simulink model "regen"  (R2024b)
settings: Solver=VariableStepAuto  StartTime=0.0  StopTime=10  FixedStep=0.001  RelTol=1e-3
settings Model: Creator=Isaac  LastModifiedBy=isaac

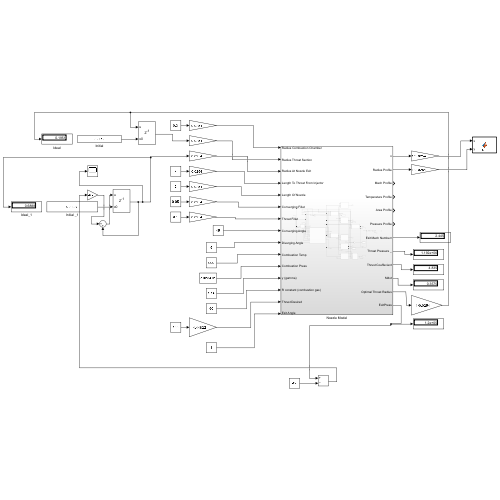
[thumbnail: Simulink's stored preview of the top-level diagram]
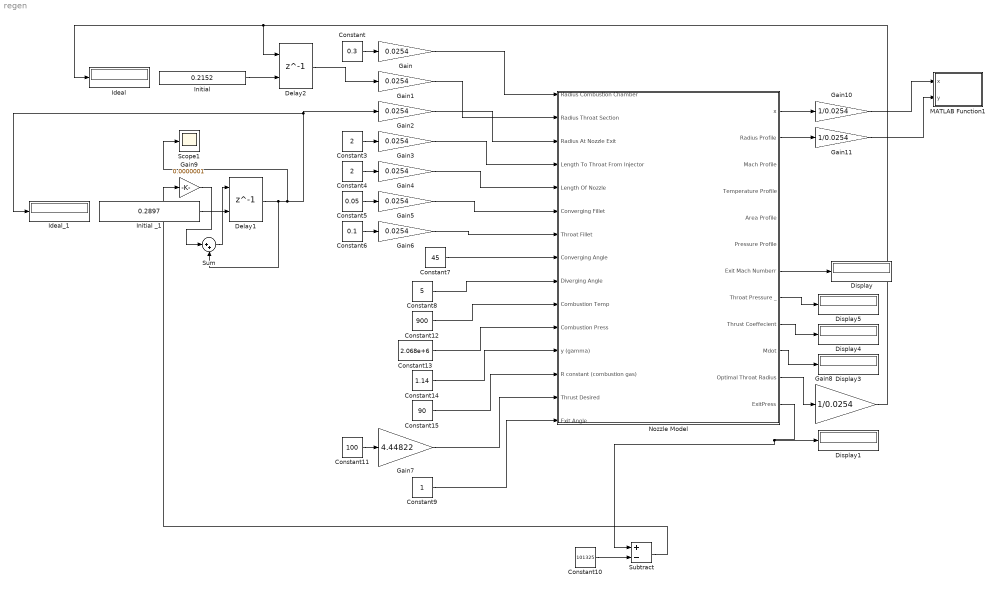
== system regen ==
  Constant : Constant  Value=0.3
  Constant10 : Constant  Value=101325
  Constant11 : Constant  Value=100
  Constant12 : Constant  Value=900
  Constant13 : Constant  Value=2.068e+6
  Constant14 : Constant  Value=1.14
  Constant15 : Constant  Value=90
  Constant3 : Constant  Value=2
  Constant4 : Constant  Value=2
  Constant5 : Constant  Value=0.05
  Constant6 : Constant  Value=0.1
  Constant7 : Constant  Value=45
  Constant8 : Constant  Value=5
  Constant9 : Constant
  Delay1 : Delay  DelayLength=1  InitialConditionSource=Input port
      settings: InputPortMap=u0,p4
  Delay2 : Delay  DelayLength=1  InitialConditionSource=Input port
      settings: InputPortMap=u0,p4
  Display{,1,3..5} (5 alike) : Display
  Gain{,1..6} (7 alike) : Gain  Gain=0.0254
  Gain10 : Gain  Gain=1/0.0254
  Gain11 : Gain  Gain=1/0.0254
  Gain7 : Gain  Gain=4.44822
  Gain8 : Gain  Gain=1/0.0254
  Gain9 : Gain  Gain=0.0000001
  Ideal : Display
  Ideal_1 : Display
  Initial : Constant  Value=0.2152
  Initial _1 : Constant  Value=0.2897
  MATLAB Function1 : MATLAB Function  TreatAsAtomicUnit=on
  Nozzle Model : Subsystem
  Scope1 : Scope
  Subtract : Sum  Inputs=+-
  Sum : Sum  Inputs=|++
  wires:
  Constant13/1 -> Nozzle Model/11(Combustion Press)
  Constant11/1 -> Gain7/1
  Constant12/1 -> Nozzle Model/10(Combustion Temp)
  Constant/1 -> Gain/1
  Constant14/1 -> Nozzle Model/12(y (gamma))
  Constant4/1 -> Gain4/1
  Constant6/1 -> Gain6/1
  Constant15/1 -> Nozzle Model/13(R constant (combustion gas))
  Constant7/1 -> Nozzle Model/8(Converging Angle)
  Constant3/1 -> Gain3/1
  Constant5/1 -> Gain5/1
  Gain4/1 -> Nozzle Model/5(Length Of Nozzle)
  Gain/1 -> Nozzle Model/1(Radius Combustion Chamber)
  Gain2/1 -> Nozzle Model/3(Radius At Nozzle Exit)
  Gain3/1 -> Nozzle Model/4(Length To Throat From Injector)
  Gain5/1 -> Nozzle Model/6(Converging Fillet)
  Gain6/1 -> Nozzle Model/7(Throat Fillet)
  Constant8/1 -> Nozzle Model/9(Diverging Angle)
  Gain7/1 -> Nozzle Model/14(Thrust Desired)
  Constant9/1 -> Nozzle Model/15(Exit Angle)
  Nozzle Model/11(Optimal Throat Radius) -> Gain8/1
  Nozzle Model/7(Exit Mach Numberr) -> Display/1
  Nozzle Model/12(ExitPress) -> Subtract/1, Display1/1
  Nozzle Model/8(Throat Pressure _) -> Display5/1
  Nozzle Model/9(Thrust Coeffecient) -> Display4/1
  Nozzle Model/10(Mdot) -> Display3/1
  Gain8/1 -> Delay2/1, Ideal/1
  Gain1/1 -> Nozzle Model/2(Radius Throat Section)
  Delay1/1 -> Sum/2, Ideal_1/1, Gain2/1, Scope1/1
  Gain9/1 -> Sum/1
  Constant10/1 -> Subtract/2
  Subtract/1 -> Gain9/1
  Sum/1 -> Delay1/1
  Initial _1/1 -> Delay1/2
  Initial/1 -> Delay2/2
  Delay2/1 -> Gain1/1
  Nozzle Model/1(x) -> Gain10/1
  Gain10/1 -> MATLAB Function1/1(x)
  Nozzle Model/2(Radius Profile) -> Gain11/1
  Gain11/1 -> MATLAB Function1/2(y)

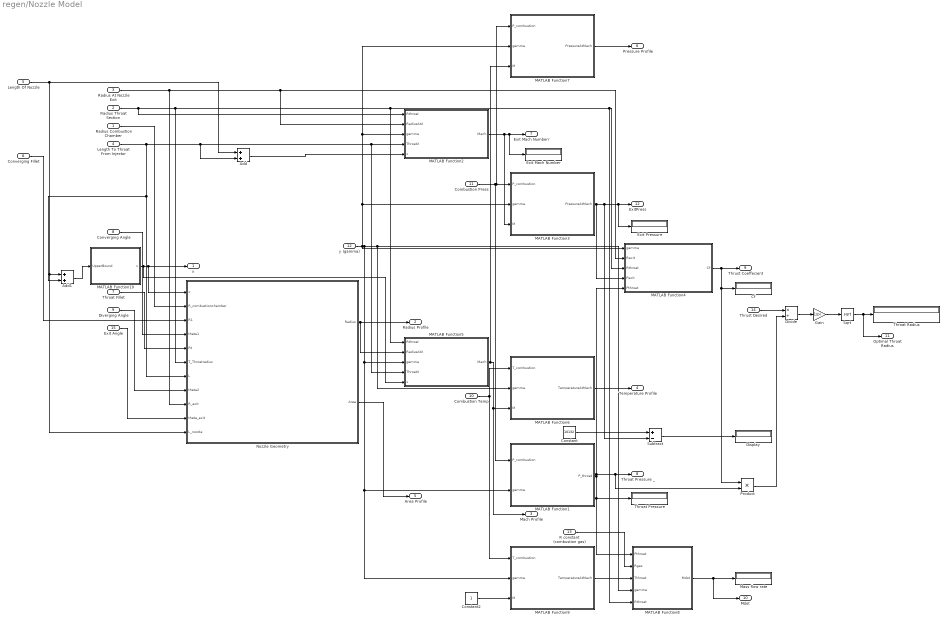
== system regen/Nozzle Model ==
  Radius Combustion Chamber : Inport
  Radius Throat Section : Inport  Port=2
  Radius At Nozzle Exit : Inport  Port=3
  Length To Throat From Injector : Inport  Port=4
  Length Of Nozzle : Inport  Port=5
  Converging Fillet : Inport  Port=6
  Throat Fillet : Inport  Port=7
  Converging Angle : Inport  Port=8
  Diverging Angle : Inport  Port=9
  Combustion Temp : Inport  Port=10
  Combustion Press : Inport  Port=11
  y (gamma) : Inport  Port=12
  R constant (combustion gas) : Inport  Port=13
  Thrust Desired : Inport  Port=14
  Exit Angle : Inport  Port=15
  Add : Sum
  Add1 : Sum
  Cf : Display
  Constant : Constant  Value=10132
  Constant2 : Constant
  Display : Display
  Divide : Product  Inputs=*/
  Exit Mach Number : Display
  Exit Pressure : Display
  Gain : Gain  Gain=1/pi
  MATLAB Function1 : MATLAB Function  TreatAsAtomicUnit=on
  MATLAB Function10 : MATLAB Function  TreatAsAtomicUnit=on
  MATLAB Function2 : MATLAB Function  TreatAsAtomicUnit=on
  MATLAB Function3 : MATLAB Function  TreatAsAtomicUnit=on
  MATLAB Function4 : MATLAB Function  TreatAsAtomicUnit=on
  MATLAB Function5 : MATLAB Function  TreatAsAtomicUnit=on
  MATLAB Function6 : MATLAB Function  TreatAsAtomicUnit=on
  MATLAB Function7 : MATLAB Function  TreatAsAtomicUnit=on
  MATLAB Function8 : MATLAB Function  TreatAsAtomicUnit=on
  MATLAB Function9 : MATLAB Function  TreatAsAtomicUnit=on
  Mass flow rate : Display
  Nozzle Geometry : MATLAB Function  TreatAsAtomicUnit=on
  Product : Product
  Sqrt : Sqrt
  Subtract : Sum  Inputs=+-
  Throat Pressure : Display
  Throat Radius : Display
  x : Outport
  Radius Profile : Outport  Port=2
  Mach Profile : Outport  Port=3
  Temperature Profile : Outport  Port=4
  Area Profile : Outport  Port=5
  Pressure Profile : Outport  Port=6
  Exit Mach Numberr : Outport  Port=7
  Throat Pressure _ : Outport  Port=8
  Thrust Coeffecient : Outport  Port=9
  Mdot : Outport  Port=10
  Optimal Throat Radius : Outport  Port=11
  ExitPress : Outport  Port=12
  wires:
  Combustion Temp/1 -> MATLAB Function6/1(T_combustion), MATLAB Function9/1(T_combustion)
  Converging Angle/1 -> Nozzle Geometry/4(theta1)
  Converging Fillet/1 -> Nozzle Geometry/3(R1)
  Length To Throat From Injector/1 -> MATLAB Function5/4(ThroatX), MATLAB Function2/4(ThroatX), Add/2, Add1/2, Nozzle Geometry/7(L)
  Combustion Press/1 -> MATLAB Function3/1(P_combustion), MATLAB Function7/1(P_combustion), MATLAB Function1/1(P_combustion)
  Diverging Angle/1 -> Nozzle Geometry/8(theta2)
  Throat Fillet/1 -> Nozzle Geometry/5(Rt)
  Length Of Nozzle/1 -> Add1/1, Nozzle Geometry/11(L_nozzle), Add/1
  Thrust Desired/1 -> Divide/1
  y (gamma)/1 -> MATLAB Function1/2(gamma), MATLAB Function9/2(gamma), MATLAB Function5/3(gamma), MATLAB Function6/2(gamma), MATLAB Function8/4(gamma), MATLAB Function7/2(gamma), MATLAB Function2/3(gamma), MATLAB Function3/2(gamma), MATLAB Function4/1(gamma)
  Add/1 -> MATLAB Function2/5(x)
  Divide/1 -> Gain/1
  Product/1 -> Divide/2
  Constant/1 -> Subtract/1
  Add1/1 -> MATLAB Function10/1(UpperBound)
  Radius At Nozzle Exit/1 -> MATLAB Function2/2(RadiusAtX), MATLAB Function4/2(Rexit), Nozzle Geometry/9(R_exit)
  Radius Combustion Chamber/1 -> Nozzle Geometry/2(R_combustionchamber)
  Radius Throat Section/1 -> MATLAB Function8/5(Rthroat), MATLAB Function4/3(Rthroat), MATLAB Function5/1(Rthroat), Nozzle Geometry/6(T_Throatradius), MATLAB Function2/1(Rthroat)
  MATLAB Function10/1(x) -> x/1, Nozzle Geometry/1(x), MATLAB Function5/5(x)
  R constant (combustion gas)/1 -> MATLAB Function8/2(Rgas)
  Exit Angle/1 -> Nozzle Geometry/10(theta_exit)
  Nozzle Geometry/1(Radius) -> Radius Profile/1, MATLAB Function5/2(RadiusAtX)
  Nozzle Geometry/2(Area) -> Area Profile/1
  MATLAB Function2/1(Mach) -> Exit Mach Numberr/1, Exit Mach Number/1, MATLAB Function3/3(M)
  Sqrt/1 -> Throat Radius/1, Optimal Throat Radius/1
  MATLAB Function5/1(Mach) -> Mach Profile/1, MATLAB Function6/3(M), MATLAB Function7/3(M)
  Constant2/1 -> MATLAB Function9/3(M)
  MATLAB Function7/1(PressureAtMach) -> Pressure Profile/1
  MATLAB Function3/1(PressureAtMach) -> ExitPress/1, Exit Pressure/1, Subtract/2, MATLAB Function4/4(Pexit)
  MATLAB Function6/1(TemperatureAtMach) -> Temperature Profile/1
  Gain/1 -> Sqrt/1
  MATLAB Function1/1(P_throat) -> Product/2, Throat Pressure _/1, MATLAB Function4/5(Pthroat), MATLAB Function8/1(Pthroat), Throat Pressure/1
  MATLAB Function9/1(TemperatureAtMach) -> MATLAB Function8/3(Tthroat)
  MATLAB Function4/1(Cf) -> Product/1, Cf/1, Thrust Coeffecient/1
  Subtract/1 -> Display/1
  MATLAB Function8/1(Mdot) -> Mass flow rate/1, Mdot/1

== matlab function regen/Nozzle Model/MATLAB Function8 ==
  data: Pthroat input; Mdot output; Rgas input; Tthroat input; gamma input; Rthroat input
function Mdot = MassFlow(Pthroat, Rgas, Tthroat, gamma, Rthroat)

Mdot = Pthroat * (Rgas * Tthroat)^-1 * sqrt(gamma * Rgas * Tthroat) * pi * Rthroat^2;

== matlab function regen/Nozzle Model/MATLAB Function9 ==
  data: T_combustion input; TemperatureAtMach output; gamma input; M input
function TemperatureAtMach = IsentropicTemperature(T_combustion, gamma, M)


TemperatureAtMach = T_combustion * (1 + 0.5*(gamma-1)*M^2)^(-1);

== matlab function regen/Nozzle Model/MATLAB Function10 ==
  data: x output size=[1 10000]; UpperBound input
function x = Span(UpperBound)

x = linspace(0, UpperBound, 10000);

== matlab function regen/MATLAB Function1 ==
  data: x input; y input
function fcn(x, y)
hold on
plot(x,y)
axis('equal')
grid on
end

== matlab function regen/Nozzle Model/Nozzle Geometry ==
  data: x input; R_combustionchamber input; R1 input; theta1 input; Rt input; T_Throatradius input; L input; theta2 input; Radius output size=[1 10000]; R_exit input; theta_exit input; L_nozzle input; Area output size=[1 10000]
function [Radius, Area] = combustionChamberProfile(x, R_combustionchamber, R1, theta1, Rt, T_Throatradius, L, theta2, R_exit, theta_exit, L_nozzle)
    y = zeros(1, length(x));
    for i=1:length(y)
    % Calculate the boundaries for each piece of the function
    boundary1 = -R1 * tan((theta1 * pi / 180) / 2) + (1 / tan(-theta1 * pi / 180)) * (R_combustionchamber + sqrt(Rt^2 - (Rt * sin(theta1 * pi / 180))^2) - T_Throatradius - Rt) + (L - Rt * sin(theta1 * pi / 180));
    
    boundary2 = boundary1 + R1 * sin(theta1 * pi / 180);
    
    boundary3 = L - Rt * sin(theta1 * pi / 180);
    
    boundary4 = L + Rt * sin(theta2 * pi / 180);
    
    exitslope = tan(theta_exit * pi / 180);

    enterslope = tan(theta2 * pi / 180);
    
    XX = [L + Rt * sin(theta2 * pi / 180), L_nozzle + L];
    YY = [-sqrt(Rt^2 - (boundary4 - L)^2) + T_Throatradius + Rt, R_exit];

    nozzleexit = spline(XX, [enterslope YY exitslope]);
    

    % Determine which piece of the function to use based on the value of x
    if x(i) >= 0 && x(i) <= boundary1
        % First piece: y = R_combustionchamber
        y(i) = R_combustionchamber;
    elseif x(i) > boundary1 && x(i) <= boundary2
        % Second piece: y = sqrt(R1^2 - (x - boundary1)^2) + R_combustionchamber - R1
        y(i) = sqrt(R1^2 - (x(i) - boundary1)^2) + R_combustionchamber - R1;
    elseif x(i) > boundary3 && x(i) <= boundary4
        % Third piece: y = -sqrt(Rt^2 - (x - L)^2) + T_Throatradius + Rt
        y(i) = -sqrt(Rt^2 - (x(i) - L)^2) + T_Throatradius + Rt;
    elseif x(i) > boundary2 && x(i) <= boundary3
        % Fourth piece: y = tan(-theta1 * pi / 180) * (x - (L - Rt * sin(theta1 * pi / 180))) - sqrt(Rt^2 - (Rt * sin(theta1 * pi / 180))^2) + T_Throatradius + Rt
        y(i) = tan(-theta1 * pi / 180) * (x(i) - (L - Rt * sin(theta1 * pi / 180))) - sqrt(Rt^2 - (Rt * sin(theta1 * pi / 180))^2) + T_Throatradius + Rt;
    elseif x(i) > boundary4 && x(i) <= XX(2)
        y(i) = ppval(nozzleexit, x(i));
    else
        % If x is outside the defined domain, return NaN (Not a Number)
        y(i) = NaN;
    end
    end

    Radius = y;
    Area = pi .* y.^2;
end

== matlab function regen/Nozzle Model/MATLAB Function1 ==
  data: P_combustion input; P_throat output; gamma input
function P_throat = ComputeThroatPressure(P_combustion, gamma)


P_throat = P_combustion*((0.5*gamma + 0.5)^((-gamma)/(gamma-1)));

== matlab function regen/Nozzle Model/MATLAB Function2 ==
  data: Rthroat input; Mach output size=1; RadiusAtX input; gamma input; ThroatX input; x input
function Mach = ComputeMach(Rthroat, RadiusAtX, gamma, ThroatX, x)



if length(x)==1
    fun = @(M) M^-2 * (2 * (gamma + 1)^-1 * (1 + 0.5*(gamma-1)*M^2))^((gamma + 1)/(gamma-1)) - (RadiusAtX/Rthroat)^2;
    if x>ThroatX
        Mach = fzero(fun, 10);
    elseif x == ThroatX
        Mach = 1;
    else
        Mach = fzero(fun, [0.001 0.9999]);
    end
else


    Mach = zeros(length(x));
    for i=1:length(Mach)
    fun = @(M) M^-2 * (2 * (gamma + 1)^-1 * (1 + 0.5*(gamma-1)*M^2))^((gamma + 1)/(gamma-1)) - (RadiusAtX(i)/Rthroat)^2;
    if x(i)>ThroatX
        Mach(i) = fzero(fun, [1.0001 10]);
    elseif x(i) == ThroatX
        Mach(i) = 1;
    else
        Mach(i) = fzero(fun, [0.001 0.9999]);
    end
    end
end

== matlab function regen/Nozzle Model/MATLAB Function3 ==
  data: P_combustion input; PressureAtMach output; gamma input; M input
function PressureAtMach = IsentropicPressure(P_combustion, gamma, M)


PressureAtMach = P_combustion .* (1 + 0.5.*(gamma-1).*M.^2).^(-gamma/(gamma-1));

== matlab function regen/Nozzle Model/MATLAB Function4 ==
  data: gamma input; Cf output; Rexit input; Rthroat input; Pexit input; Pthroat input
function Cf = ThrustCoeff(gamma, Rexit, Rthroat, Pexit, Pthroat)

Cf = sqrt(2 * gamma ^2 * (gamma-1)^-1 * (0.5*(gamma+1))^((gamma+1)/(gamma-1)) * (1-(Pexit/Pthroat)^((gamma-1)/gamma))) + (Rexit/Rthroat)^2 * (Pexit/Pthroat);

== matlab function regen/Nozzle Model/MATLAB Function5 ==
  data: Rthroat input; Mach output size=[1 10000]; RadiusAtX input; gamma input; ThroatX input; x input
function Mach = ComputeMach(Rthroat, RadiusAtX, gamma, ThroatX, x)


Mach = zeros(1,length(x));
for i=1:length(Mach)
fun = @(M) M^-2 * (2 * (gamma + 1)^-1 * (1 + 0.5*(gamma-1)*M^2))^((gamma + 1)/(gamma-1)) - (RadiusAtX(i)/Rthroat)^2;
if x(i)>ThroatX
    Mach(i) = fzero(fun, 10);
elseif x(i) == ThroatX
    Mach(i) = 1;
else
    Mach(i) = fzero(fun, 0.5);
end
end

== matlab function regen/Nozzle Model/MATLAB Function6 ==
  data: T_combustion input; TemperatureAtMach output size=[1 10000]; gamma input; M input
function TemperatureAtMach = IsentropicTemperature(T_combustion, gamma, M)


TemperatureAtMach = T_combustion .* (1 + 0.5.*(gamma-1).*M.^2).^(-1);

== matlab function regen/Nozzle Model/MATLAB Function7 ==
  data: P_combustion input; PressureAtMach output size=[1 10000]; gamma input; M input
function PressureAtMach = IsentropicPressure(P_combustion, gamma, M)


PressureAtMach = P_combustion .* (1 + 0.5.*(gamma-1).*M.^2).^(-gamma/(gamma-1));
